simulink model "bball_learned_HA0"  (R2022b)
settings: Solver=FixedStepAuto  StartTime=0.0  StopTime=timeFinal  FixedStep=timeStepMax  RelTol=1e-3
undefined symbols (not defined in the file): a1, a2
settings Model: Creator=jun  LastModifiedBy=jun

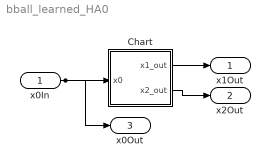
== system bball_learned_HA0 ==
  x0In : Inport
  Chart : Stateflow chart  TreatAsAtomicUnit=on
  x1Out : Outport  SignalName=x1Out
  x2Out : Outport  Port=2  SignalName=x2Out
  x0Out : Outport  Port=3  SignalName=x0Out
  wires:
  Chart/2(x2_out) -> x2Out/1
  Chart/1(x1_out) -> x1Out/1
  x0In/1 -> x0Out/1, Chart/1(x0)

== stateflow chart bball_learned_HA0/Chart ==
  settings: updateMethod=CONTINUOUS  executeAtInitialization=1
  state loc1
    du:
    x1_dot = x0 * 1.439521602522647e-09 + x1 * -3.3857767978151543e-10 + x2 * 0.9999999999763148 + 1.4714478913102624e-08;
    x2_dot = x0 * 1.0000011406940934 + x1 * -2.7325120076807296e-07 + x2 * -7.44550887279102e-08 + 1.4448547477246617e-05;
    exit:
    x1_out = x1;
    x2_out = x2;
  (junction 2) -> loc1 : [x0 * 0.0024183437554309785 + x1 * 7.0612063150346565 + x2 * 0.00969564568453575 + -0.9371314133763816 <= 0]{x1 = x0 * 0.0 + x1 * 0.0 + x2 * 0.0 + 0.0; x2 = x0 * 6.351585073558323e-15 + x1 * -4.862776847858186e-13 + x2 * -0.8000000000000029 + 6.394884621840902e-14; }
  (default) -> loc1 : { x1 = a1; x2 = a2; }
  loc1 -> (junction 5) [order 2]
  (junction 5) -> loc1 : { x1 = x1; x2 = x2; }
  loc1 -> (junction 2) [order 1]
  data: x0 input; x1_out output; x2_out output; x1 local double; x2 local double; a1 parameter; a2 parameter
  data x1 settings: updateMethod=SF_CONTINUOUS_TIME_DATA
  data x2 settings: updateMethod=SF_CONTINUOUS_TIME_DATA
